simulink model "Wiring_Diagram_Simulink"  (R2026a)
settings: Solver=VariableStepAuto
settings Model: Creator=lewis  LastModifiedBy=lewis
settings DebuggingCC: MergeDetectMultiDrivingBlocksExec=error
settings ModelReferenceCC: PropagateSignalLabelsOutOfModel=on

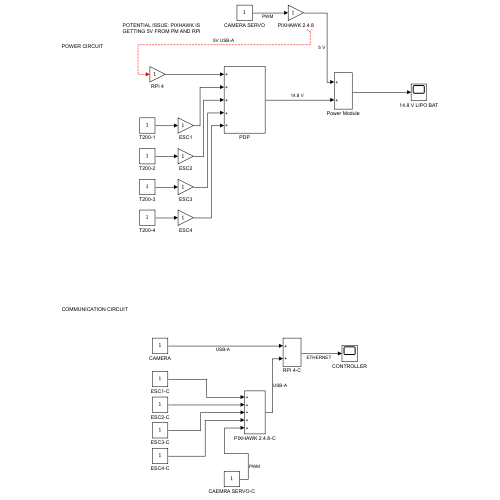
[thumbnail: Simulink's stored preview of the top-level diagram]
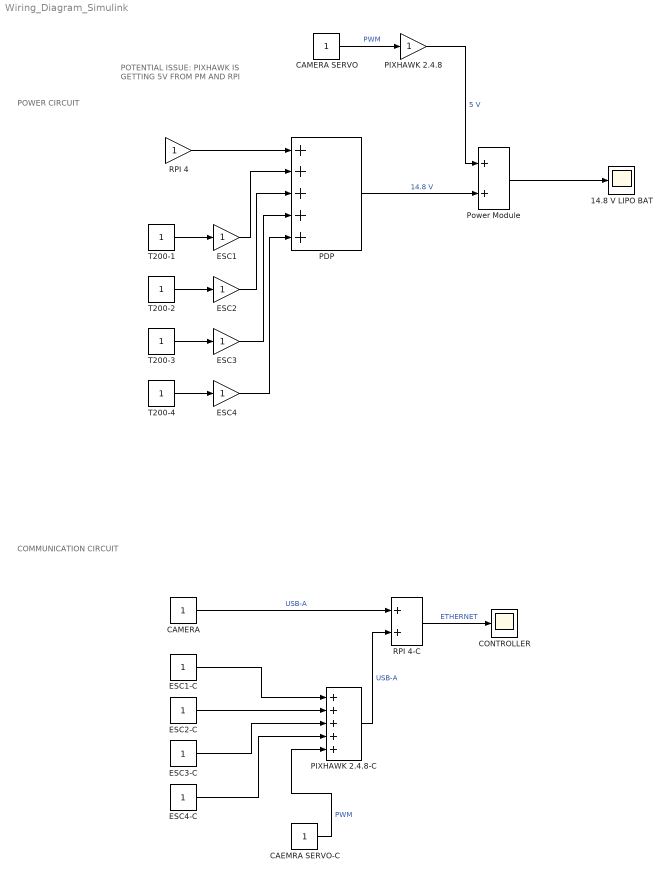
== system Wiring_Diagram_Simulink ==
  note: POTENTIAL ISSUE: PIXHAWK IS GETTING 5V FROM PM AND RPI
  note: COMMUNICATION CIRCUIT
  note: POWER CIRCUIT
  14.8 V LIPO BAT : Scope
  CAEMRA SERVO-C : Constant
  CAMERA : Constant
  CAMERA SERVO : Constant
  CONTROLLER : Scope
  ESC{1..4} (4 alike) : Gain
  ESC1-C : Constant
  ESC2-C : Constant
  ESC3-C : Constant
  ESC4-C : Constant
  PDP : Sum  Inputs=+++++
  PIXHAWK 2.4.8 : Gain
  PIXHAWK 2.4.8-C : Sum  Inputs=+++++
  Power Module : Sum
  RPI 4 : Gain
  RPI 4-C : Sum
  T200-{1..4} (4 alike) : Constant
  wires:
  PDP/1 -> Power Module/2  "14.8 V"
  Power Module/1 -> 14.8 V LIPO BAT/1
  T200-1/1 -> ESC1/1
  ESC1/1 -> PDP/2
  T200-2/1 -> ESC2/1
  ESC2/1 -> PDP/3
  ESC3/1 -> PDP/4
  T200-3/1 -> ESC3/1
  T200-4/1 -> ESC4/1
  PIXHAWK 2.4.8/1 -> Power Module/1  "5 V"
  CAMERA SERVO/1 -> PIXHAWK 2.4.8/1  "PWM"
  RPI 4/1 -> PDP/1
  ESC4/1 -> PDP/5
  PIXHAWK 2.4.8-C/1 -> RPI 4-C/2  "USB-A"
  ESC1-C/1 -> PIXHAWK 2.4.8-C/1
  ESC2-C/1 -> PIXHAWK 2.4.8-C/2
  ESC3-C/1 -> PIXHAWK 2.4.8-C/3
  ESC4-C/1 -> PIXHAWK 2.4.8-C/4
  CAEMRA SERVO-C/1 -> PIXHAWK 2.4.8-C/5  "PWM"
  RPI 4-C/1 -> CONTROLLER/1  "ETHERNET"
  CAMERA/1 -> RPI 4-C/1  "USB-A"
  ? -> RPI 4/1  "5V USB-A"
